simulink subsystem "PM100DXR_MC"  (R2023b)
settings: Solver=VariableStepAuto  StartTime=0.0  StopTime=10.0  RelTol=1e-3
undefined symbols (not defined in the file or in its folder): canChannel
libraries: canlib x4, canmsglib x2
settings Model: Creator=diego  LastModifiedBy=mjmag

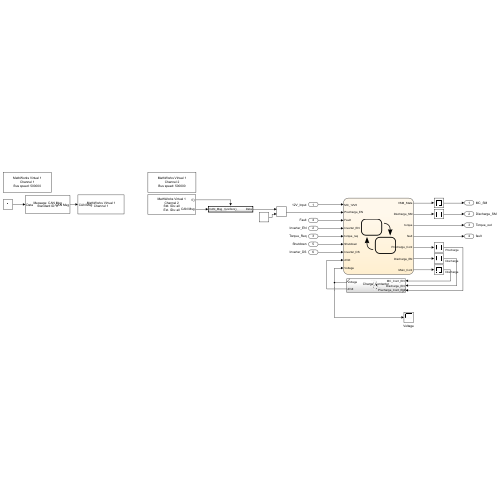
[thumbnail: Simulink's stored preview of the top-level diagram]
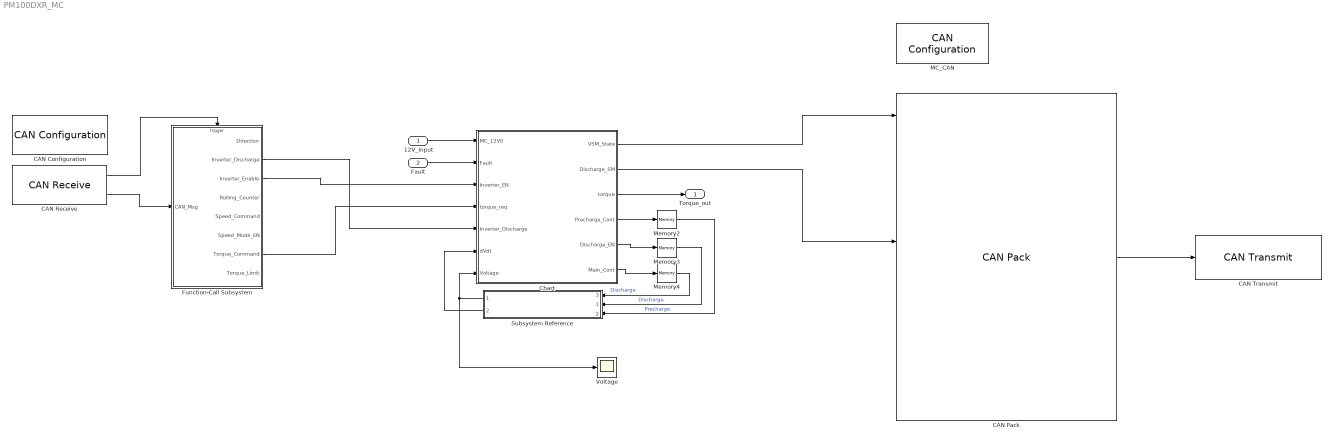
== system PM100DXR_MC ==
  12V_Input : Inport
  Fault : Inport  Port=2
  CAN Configuration : canlib/CAN Configuration  BlockHandle=6466.0006  Device=MathWorks Virtual 1 (Channel 2)  DeviceMenu=MathWorks Virtual 1 (Channel 2)  ObjConstructor=canChannel('MathWorks', 'Virtual 1', 2)  BusSpeed=500000  EnableBitParameters=off  AckMode=Normal
  CAN Pack : canmsglib/CAN Pack  CANdbFile=C:\Users\mjmag\CLionProjects\VCU-model\Powertrain_CAN.dbc  MsgList=M170_Internal_States  MsgName=M170_Internal_States  MsgIDType=Standard (11-bit identifier)  MsgIdentifier=170  MsgLength=8  Remote=off  ApplyMinMax=off  BusOutput=off  SignalInfo={'D1_PWM_Frequency','8','8','LE','unsigned','Standard','0','1','0','0','255';'D1_VSM_State','0','8','LE','unsigned','Standard','0','1','0','0','15';'D2_Inverter_State','16','8','LE','unsigned','Standard','0','1','0','0','255';'D3_Relay_1_Status','24','1','LE','unsigned','Standard','0','1','0','0','1';'D3_Relay_2_Status','25','1','LE','unsigned','Standard','0','1','0','0','1';'D3_Relay_3_Status','26','1','LE','unsigned','Standard','0','1','0','0','1';'D3_Relay_4_Status','27','1','LE','unsigned','Standard','0','1','0','0','1';'D3_Relay_5_Status','28','1','LE','unsigned','Standard','0','1','0','0','1';'D3_Relay_6_Status','29','1','LE','unsigned','Standard','0','1','0','0','1';'D4_Inverter_Discharge_State','37','3','LE','unsigned','Standard','0','1','0','0','7';'D4_Inverter_Run_Mode','32','1','LE','unsigned','Standard','0','1','0','0','1';'D5_Inverter_Command_Mode','40','1','LE','unsigned','Standard','0','1','0','0','1';'D5_Rolling_Counter','44','4','LE','unsigned','Standard','0','1','0','0','15';'D6_Inverter_Enable_Lockout','55','1','LE','unsigned','Standard','0','1','0','0','1';'D6_Inverter_Enable_State','48','1','LE','unsigned','Standard','0','1','0','0','1';'D6_Start_Mode_Active','54','1','LE','unsigned','Standard','0','1','0','0','1';'D7_BMS_Active','57','1','LE','unsigned','Standard','0','1','0','0','1';'D7_BMS_Torque_Limiting','58','1','LE','unsigned','Standard','0','1','0','0','1';'D7_Direction_Command','56','1','LE','unsigned','Standard','0','1','0','0','1';'D7_Low_Speed_Limiting','61','1','LE','unsigned','Standard','0','1','0','0','1';'D7_Max_Speed_Limiting','59','1','LE','unsigned','Standard','0','1','0','0','1'}
      settings: LibrarySourceBlock=canlib/CAN Pack  DataFormat=CANdb specified signals
  CAN Receive : canlib/CAN Receive  BlockHandle=6468.0001  Device=MathWorks Virtual 1 (Channel 2)  DeviceMenu=MathWorks Virtual 1 (Channel 2)  ObjConstructor=canChannel('MathWorks', 'Virtual 1', 2)  EnableStandardIDsFilter=off  StdIDsCombo=Allow only  StandardIDs=192  EnableExtendedIDsFilter=off  ExtIDsCombo=Allow all  ExtendedIDs=0  SampleTime=0.01  MsgsPerTimestep=all  InternalFilterUpdateStatus=on  BusOutput=off
  CAN Transmit : canlib/CAN Transmit  BlockHandle=6469.0001  Device=MathWorks Virtual 1 (Channel 1)  DeviceMenu=MathWorks Virtual 1 (Channel 1)  ObjConstructor=canChannel('MathWorks', 'Virtual 1', 1)  EnableEventTransmit=off  EnablePeriodicTransmit=off  MessagePeriod=1.000
  Chart : Stateflow chart  TreatAsAtomicUnit=on
      settings: PortSchema="{\"entries\":[{\"content\":{\"sides\":[{\"content\":{\"connectorIds\":[\"In3\",\"In1\",\"In2\",\"In6\",\"In4\",\"In7\",\"In5\"]},\"type\":\"ConnectorPlacement.EquallySpacedRectSide\",\"uuid\":\"03599179-c40e-45c0-8f83-03707e7643a9\"},{\"content\":{\"connectorIds\":[\"Out1\",\"Out2\",\"Out6\",\"Out3\",\"Out4\",\"Out5\"],\"side\":\"RIGHT\"},\"type\":\"ConnectorPlacement.EquallySpacedRectSide\",\"uuid\":\"77c27c81-6b7f-49bb-b8ad-65b312eda7e2\"},{\"content\":{\"side\":\"TOP\"},\"type\":\"ConnectorPlacement.EquallySpacedRectSide\",\"uuid\":\"12a0a04d-7874-431f-b4d8-e9223037e866\"}]},\"type\":\"ConnectorPlacement.EquallySpacedConnector\",\"uuid\":\"58e614a8-4325-4fa7-852b-761998465240\"}],\"packageUris\":[\"http://schema.mathworks.com/mf0/Connector/R2020b\"],\"version\":\"1.0\"}"
  Function-Call Subsystem : Subsystem  TreatAsAtomicUnit=on
  MC_CAN : canlib/CAN Configuration  BlockHandle=6523.0001  Device=MathWorks Virtual 1 (Channel 1)  DeviceMenu=MathWorks Virtual 1 (Channel 1)  ObjConstructor=canChannel('MathWorks', 'Virtual 1', 1)  BusSpeed=500000  EnableBitParameters=off  AckMode=Normal
  Memory2 : Memory
  Memory3 : Memory
  Memory4 : Memory
  Subsystem Reference : Subsystem  ReferencedSubsystem=Charge_Contactor
      settings: PortSchema="{\"entries\":[{\"content\":{\"sides\":[{\"content\":{\"connectorIds\":[\"In3\",\"In1\",\"In2\"]},\"type\":\"ConnectorPlacement.EquallySpacedRectSide\",\"uuid\":\"c4a26b2a-75b7-46e9-83ad-f08a209eb654\"},{\"content\":{\"connectorIds\":[\"Out1\",\"Out2\"],\"side\":\"RIGHT\"},\"type\":\"ConnectorPlacement.EquallySpacedRectSide\",\"uuid\":\"e0e23db8-3606-4757-a6fd-db7c1d3e8c5a\"},{\"content\":{\"side\":\"TOP\"},\"type\":\"ConnectorPlacement.EquallySpacedRectSide\",\"uuid\":\"0a967cd1-2252-4813-adc7-d3e8433b462a\"}]},\"type\":\"ConnectorPlacement.EquallySpacedConnector\",\"uuid\":\"d4c2dd3c-9ab6-4575-a91c-d1aa35d96284\"}],\"packageUris\":[\"http://schema.mathworks.com/mf0/Connector/R2020b\"],\"version\":\"1.0\"}"
  Voltage : Scope
  Torque_out : Outport
  wires:
  Chart/3(Precharge_Cont) -> Memory2/1
  Fault/1 -> Chart/1(Fault)
  Subsystem Reference/1 -> Chart/5(Voltage), Voltage/1
  12V_Input/1 -> Chart/3(MC_12V0)
  Chart/1(VSM_State) -> CAN Pack/2
  Function-Call Subsystem/2(Inverter_Discharge) -> Chart/4(Inverter_Discharge)
  Chart/4(Discharge_EN) -> Memory3/1
  Memory3/1 -> Subsystem Reference/1  "Discharge"
  Memory2/1 -> Subsystem Reference/2  "Precharge"
  Function-Call Subsystem/7(Torque_Command) -> Chart/6(torque_req)
  Chart/6(torque) -> Torque_out/1
  Subsystem Reference/2 -> Chart/7(dVdt)
  Chart/5(Main_Cont) -> Memory4/1
  Memory4/1 -> Subsystem Reference/3  "Discharge"
  CAN Receive/2 -> Function-Call Subsystem/1(CAN_Msg)
  CAN Receive/1 -> Function-Call Subsystem/Trigger
  Function-Call Subsystem/3(Inverter_Enable) -> Chart/2(Inverter_EN)
  Chart/2(Discharge_SM) -> CAN Pack/10
  CAN Pack/1 -> CAN Transmit/1

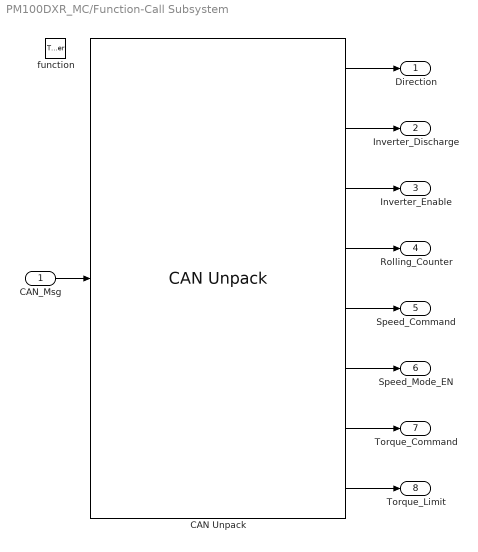
== system PM100DXR_MC/Function-Call Subsystem ==
  CAN_Msg : Inport
  function : TriggerPort  TriggerType=function-call  VariantControl=(inherit)
  CAN Unpack : canmsglib/CAN Unpack  CANdbFile=C:\Users\heyka\MATLAB\Projects\VCU_C\MC_CAN.dbc  MsgList=(none)  MsgName=M192_Command_Message  MsgIDType=Standard (11-bit identifier)  MsgIdentifier=192  MsgLength=8  SignalInfo={'Direction_Command','32','1','LE','unsigned','Standard','0','1','0','0','1';'Inverter_Discharge','41','1','LE','unsigned','Standard','0','1','0','0','1';'Inverter_Enable','40','1','LE','unsigned','Standard','0','1','0','0','1';'RollingCounter','44','4','LE','unsigned','Standard','0','1','0','0','15';'Speed_Command','16','16','LE','signed','Standard','0','1','0','-32768','32767';'Speed_Mode_Enable','42','1','LE','unsigned','Standard','0','1','0','0','1';'Torque_Command','0','16','LE','signed','Standard','0','0.1','0','-3276.8','3276.7';'Torque_Limit_Command','48','16','LE','signed','Standard','0','0.1','0','-3276.8','3276.7'}  IDPort=off  TimestampPort=off  ErrorPort=off  RemotePort=off  LengthPort=off  StatusPort=off  ApplyMinMax=off
      settings: DataFormat=CANdb specified signals
  Direction : Outport
  Inverter_Discharge : Outport  Port=2
  Inverter_Enable : Outport  Port=3
  Rolling_Counter : Outport  Port=4
  Speed_Command : Outport  Port=5
  Speed_Mode_EN : Outport  Port=6
  Torque_Command : Outport  Port=7
  Torque_Limit : Outport  Port=8
  wires:
  CAN Unpack/8 -> Torque_Limit/1
  CAN Unpack/7 -> Torque_Command/1
  CAN Unpack/6 -> Speed_Mode_EN/1
  CAN Unpack/5 -> Speed_Command/1
  CAN Unpack/3 -> Inverter_Enable/1
  CAN Unpack/4 -> Rolling_Counter/1
  CAN Unpack/2 -> Inverter_Discharge/1
  CAN_Msg/1 -> CAN Unpack/1
  CAN Unpack/1 -> Direction/1

== stateflow chart PM100DXR_MC/Chart ==
  state Motor_Controller
    state Power_ON
      entry:
      VSM_State = 0;
      Discharge_SM = 0;
    state Precharge
      entry:
      VSM_State = 1;
      Discharged = 0;
      state Precharge2
        during:
        VSM_State = 3;
        dV = dVdt
      state Precharge3
        entry:
        VSM_State = 4;
        Precharge_Cont = 0;
        Main_Cont = 1;
      state Precharge1
        during:
        VSM_State = 2;
        dV = 1000;
        Precharge_Cont = 1;
      (default) -> Precharge1
      Precharge1 -> Precharge2 : [dV ~= dVdt]
      Precharge2 -> Precharge3 : [dV<56]
    state Fault
      entry:
      VSM_State = 9;
    state Running
      entry:
      VSM_State = 6;
      during:
      torque = torque_req;
      exit:
      torque = 0;
    state Ready
      entry:
      VSM_State = 5;
    state Shutdown
      entry:
      VSM_State = 14;
      Discharge_EN = 0;
      Discharged = 1;
    state Discharge
      entry:
      VSM_State = 7;
      Main_Cont = 0;
      state Discharge1
        entry:
        Discharge_SM = 1;
        Discharge_EN = 1;
      state Discharge2
        entry:
        Discharge_SM = 2;
      state Discharge4
        entry:
        Discharge_SM = 4;
      state Discharge3
        entry:
        Discharge_SM = 3;
      (default) -> Discharge1
      Discharge1 -> Discharge2
      Discharge2 -> Discharge3 : [RPM < 75]
      Discharge3 -> Discharge4 : [ Voltage < 30]
    (default) -> Power_ON
    Shutdown -> Power_ON : [MC_12V0 <= 1]
    Power_ON -> Precharge : [MC_12V0 >= 1]
    Precharge3 -> Ready
    Motor_Controller -> Fault [order 2] : [Fault ==1  && Discharge_EN ~= 1 && MC_12V0 > 1]
    Ready -> Running : [Inverter_EN == 1 && torque_req == 0]
    Running -> Ready : [Inverter_EN == 0]
    Fault -> Discharge : [MC_12V0 <= 1]
    Discharge -> Shutdown : [Discharge_SM == 4]
    Motor_Controller -> Discharge [order 1] : [Inverter_Discharge == 1 && VSM_State ~= 7 && Discharged == 0]
  (default) -> Motor_Controller
  data: Fault input; VSM_State output [0..14] =0; Inverter_EN input; Discharge_SM output =1; RPM local =0; MC_12V0 input; Inverter_Discharge input; Precharge_Cont output; Voltage input =0; Discharge_EN output =0; Main_Cont output =0; torque_req input; torque output; dVdt input; dV local =1000; Discharged local =1
